simulink model "laborator_03"  (R2023b)
settings: Solver=VariableStepAuto  StartTime=0.0  StopTime=50  MaxStep=1e-3  RelTol=1e-3
settings Model: Creator=ovidiuceoca  LastModifiedBy=ovidiuceoca

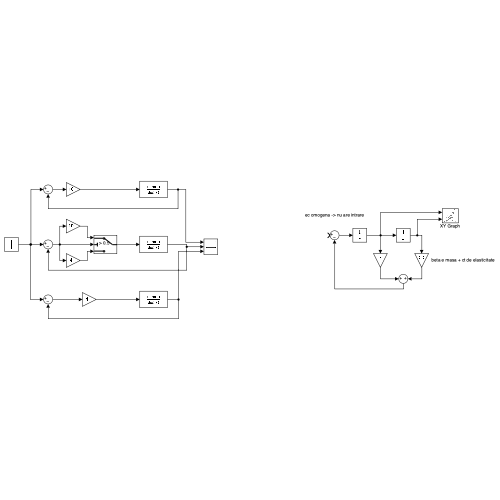
[thumbnail: Simulink's stored preview of the top-level diagram]
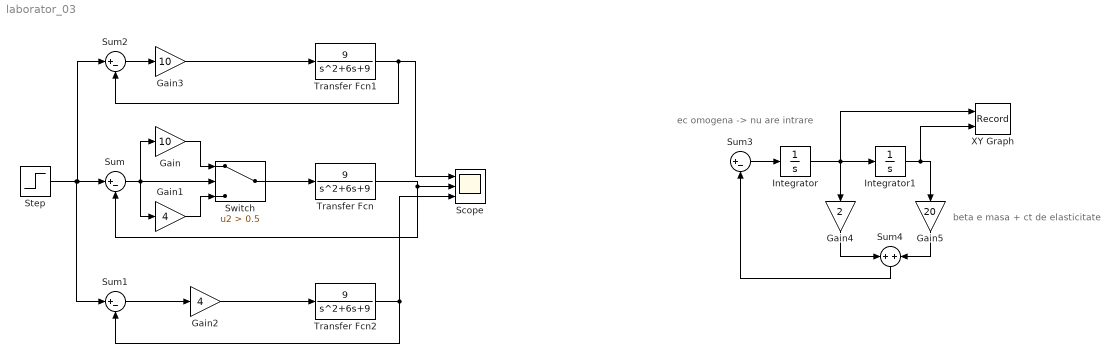
== system laborator_03 ==
  note: beta e masa + ct de elasticitate
  note: ec omogena -> nu are intrare
  Gain : Gain  Gain=10
  Gain1 : Gain  Gain=4
  Gain2 : Gain  Gain=4
  Gain3 : Gain  Gain=10
  Gain4 : Gain  Gain=2
  Gain5 : Gain  Gain=20
  Integrator : Integrator  InitialCondition=3
  Integrator1 : Integrator  InitialCondition=5
  Scope : Scope  NumInputPorts=3
  Step : Step  Time=0  SampleTime=0
  Sum{,1..3} (4 alike) : Sum  Inputs=|+-
  Sum4 : Sum  Inputs=+|+
  Switch : Switch  Criteria=u2 > Threshold  Threshold=0.5  SaturateOnIntegerOverflow=off  InputSameDT=off
  Transfer Fcn : TransferFcn  Numerator=[9]  Denominator=[1 6 9]
  Transfer Fcn1 : TransferFcn  Numerator=[9]  Denominator=[1 6 9]
  Transfer Fcn2 : TransferFcn  Numerator=[9]  Denominator=[1 6 9]
  XY Graph : Record  FileSettingsInternal="{\"entries\":[{\"content\":{\"excelSettings\":{\"content\":{},\"type\":\"Streamout.ExcelSettings\"}},\"type\":\"Streamout.FileSettingStorage\",\"uuid\":\"\"}],\"packageUris\":[\"http:\\/\\/schema.mathworks.com\\/mf0\\/streamout_blocks\\/R2020a\"],\"version\":\"1.0\"}"  Layout=[1 1]  SignalsInternal="{\"entries\":[{\"content\":{\"signals\":[{\"content\":{\"blockPath\":[],\"dimensions\":[1],\"domain\":\"\",\"lineColor\":\"#a2142f\",\"plots\":[1],\"port\":1,\"sid\":[\"\"],\"signalID\":281,\"signalName\":\"Integrator\"},\"type\":\"RecordBlkView.Signal\",\"uuid\":\"\"},{\"content\":{\"blockPath\":[],\"dimensions\":[1],\"domain\":\"\",\"lineColor\":\"#139fff\",\"plots\":[1],\"port\":2,\"sid\":[\"\"],\"signalID\":285,\"signalName\":\"Integrator1\"},\"type\":\"RecordBlkView.Signal\",\"uuid\":\"\"}]},\"type\":\"RecordBlkView.InputSignals\",\"uuid\":\"\"}],\"packageUris\":[\"http:\\/\\/schema.mathworks.com\\/mf0\\/streamout_blocks\\/R2020a\"],\"version\":\"1.0\"}"  VisualizationBindings="{\"xyplotplugin\":{\"info\":[{\"series\":[{\"bindingParametersList\":[{\"parameter\":\"X-Axis\",\"signalID\":281,\"signalName\":\"Integrator\"},{\"parameter\":\"Y-Axis\",\"signalID\":285,\"signalName\":\"Integrator1\"}],\"seriesID\":2632}],\"subplotID\":1}]}}"  CompatibilityTag=XY
  wires:
  Step/1 -> Sum2/1, Sum/1, Sum1/1
  Sum/1 -> Gain1/1, Gain/1, Switch/2
  Gain1/1 -> Switch/3
  Gain/1 -> Switch/1
  Switch/1 -> Transfer Fcn/1
  Transfer Fcn/1 -> Sum/2, Scope/2
  Sum1/1 -> Gain2/1
  Gain2/1 -> Transfer Fcn2/1
  Transfer Fcn2/1 -> Scope/3, Sum1/2
  Sum2/1 -> Gain3/1
  Gain3/1 -> Transfer Fcn1/1
  Transfer Fcn1/1 -> Sum2/2, Scope/1
  Integrator/1 -> XY Graph/1, Integrator1/1, Gain4/1
  Integrator1/1 -> XY Graph/2, Gain5/1
  Sum3/1 -> Integrator/1
  Gain4/1 -> Sum4/1
  Gain5/1 -> Sum4/2
  Sum4/1 -> Sum3/2
